simulink library "simpleDragTurbine_ul"  (R2018b)
settings: Solver=VariableStepAuto  StartTime=0.0  StopTime=10.0  RelTol=1e-3
values from neighbouring files (symbols this model uses):
  rho_fluid = 1    [simpleDragTurbine_ts.m]
undefined symbols (not defined in the file or in its folder): turbine
libraries: vrlib x1, eulAng2RotMat_ul x1, vectorDirection x1
settings Model: Creator=Ayaz  LastModifiedBy=asiddiq2

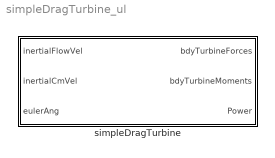
== system simpleDragTurbine_ul ==
  simpleDragTurbine : Subsystem  TreatAsAtomicUnit=on  mask{rho_fluid=rho_fluid, turb_struct=turbine}
      mask prompts: rho_fluid "Fluid density"; turb_struct "Turbines structure"

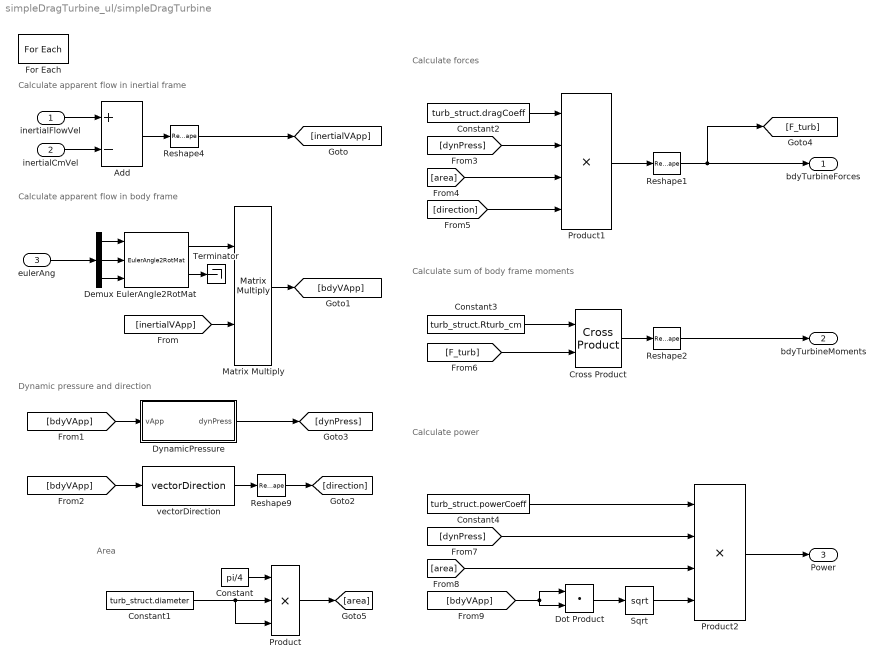
== system simpleDragTurbine_ul/simpleDragTurbine ==
  note: Calculate apparent flow in inertial frame
  note: Area
  note: Calculate apparent flow in body frame
  note: Calculate forces
  note: Calculate power
  note: Dynamic pressure and direction
  note: Calculate sum of body frame moments
  inertialFlowVel : Inport
  inertialCmVel : Inport  Port=2
  eulerAng : Inport  Port=3
  Add : Sum  Inputs=+-
  Constant : Constant  Value=pi/4
  Constant1 : Constant  Value=turb_struct.diameter  VectorParams1D=off
  Constant2 : Constant  Value=turb_struct.dragCoeff  VectorParams1D=off
  Constant3 : Constant  Value=turb_struct.Rturb_cm  VectorParams1D=off
  Constant4 : Constant  Value=turb_struct.powerCoeff  VectorParams1D=off
  Cross Product : vrlib/Utilities/Cross Product
      settings: SourceProductBaseCode=VR
  Demux : Demux  Outputs=3
  Dot Product : DotProduct  InputSameDT=on  OutDataTypeStr=Inherit: Inherit via internal rule
  DynamicPressure : Subsystem  mask{rho=rho_fluid}
      mask prompts: rho "Fluid density"
  EulerAngle2RotMat : eulAng2RotMat_ul/EulerAngle2RotMat  SystemSampleTime=-1
  For Each : ForEach  DisableCoverage=on  IterateSubsysMaskParameter=off,on  SubsysMaskParameterIterationDimension=1,2  IndexMode=One-based
  Matrix Multiply : Product  Multiplication=Matrix(*)
  Product : Product  Inputs=3
  Product1 : Product  Inputs=4
  Product2 : Product  Inputs=4
  Reshape{1..2,4,9} (4 alike) : Reshape  OutputDimensionality=Column vector (2-D)
  Sqrt : Sqrt  SaturateOnIntegerOverflow=on
  Terminator : Terminator
  vectorDirection : vectorDirection/vectorDirection  SystemSampleTime=-1
  bdyTurbineForces : Outport  PortDimensions=[3,1]  ConcatenationDimension=2
  bdyTurbineMoments : Outport  Port=2  PortDimensions=[3,1]  ConcatenationDimension=2
  Power : Outport  Port=3  PortDimensions=[1,1]  ConcatenationDimension=2
  wires:
  inertialCmVel/1 -> Add/2
  inertialFlowVel/1 -> Add/1
  DynamicPressure/1(dynPress) -> [dynPress]
  vectorDirection/1 -> Reshape9/1
  Matrix Multiply/1 -> [bdyVApp]
  [bdyVApp] -> DynamicPressure/1(vApp)
  EulerAngle2RotMat/2 -> Terminator/1
  eulerAng/1 -> Demux/1
  Demux/3 -> EulerAngle2RotMat/3
  EulerAngle2RotMat/1 -> Matrix Multiply/1
  Demux/2 -> EulerAngle2RotMat/2
  Demux/1 -> EulerAngle2RotMat/1
  [bdyVApp] -> vectorDirection/1
  [inertialVApp] -> Matrix Multiply/2
  Cross Product/1 -> Reshape2/1
  Constant/1 -> Product/1
  Product/1 -> [area]
  Product1/1 -> Reshape1/1
  Product2/1 -> Power/1
  Add/1 -> Reshape4/1
  Reshape4/1 -> [inertialVApp]
  Reshape9/1 -> [direction]
  Constant1/1 -> Product/3, Product/2
  Constant2/1 -> Product1/1
  [dynPress] -> Product1/2
  [area] -> Product1/3
  [direction] -> Product1/4
  Constant3/1 -> Cross Product/1
  [F_turb] -> Cross Product/2
  [area] -> Product2/3
  [dynPress] -> Product2/2
  Constant4/1 -> Product2/1
  [bdyVApp] -> Dot Product/1, Dot Product/2
  Dot Product/1 -> Sqrt/1
  Sqrt/1 -> Product2/4
  Reshape1/1 -> bdyTurbineForces/1, [F_turb]
  Reshape2/1 -> bdyTurbineMoments/1

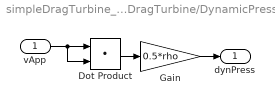
== system simpleDragTurbine_ul/simpleDragTurbine/DynamicPressure ==
  vApp : Inport
  Dot Product : DotProduct  InputSameDT=on  OutDataTypeStr=Inherit: Inherit via internal rule
  Gain : Gain  Gain=0.5*rho
  dynPress : Outport
  wires:
  Gain/1 -> dynPress/1
  vApp/1 -> Dot Product/2, Dot Product/1
  Dot Product/1 -> Gain/1
